simulink model "MobileRobotController"  (R2021b)
settings: Solver=VariableStepAuto  StartTime=0.0  StopTime=10.0  RelTol=1e-3
libraries: mobileRoboticsLib x3
settings Model: Creator=EarthPhisek  LastModifiedBy=EarthPhisek

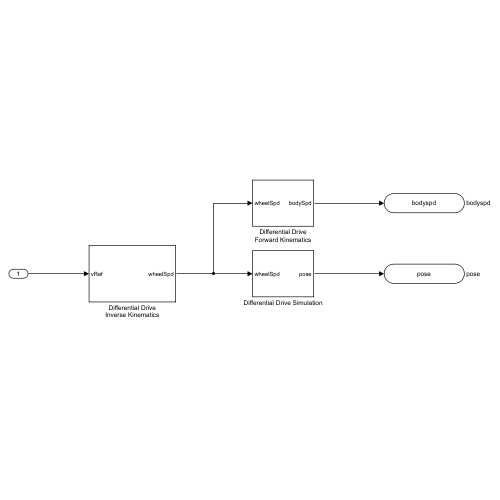
[thumbnail: Simulink's stored preview of the top-level diagram]
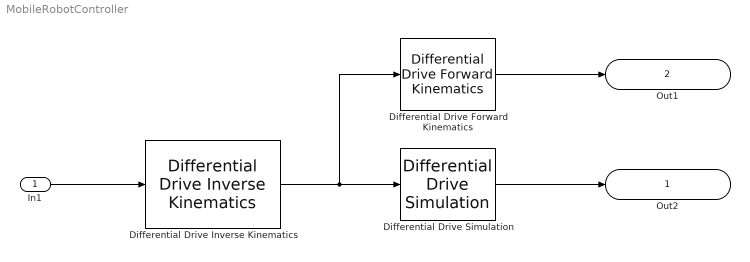
== system MobileRobotController ==
  In1 : Inport
  Differential Drive Forward Kinematics : mobileRoboticsLib/Kinematic Models/Differential Drive/Differential Drive Forward Kinematics  wheelRadius=0.1  wheelBase=0.5
      settings: SourceProductName=Mobile Robotics Simulation Toolbox
  Differential Drive Inverse Kinematics : mobileRoboticsLib/Kinematic Models/Differential Drive/Differential Drive Inverse Kinematics  wheelRadius=0.1  wheelBase=0.5
      settings: SourceProductName=Mobile Robotics Simulation Toolbox
  Differential Drive Simulation : mobileRoboticsLib/Kinematic Models/Differential Drive/Differential Drive Simulation  wheelRadius=0.1  wheelBase=0.5  initX=0  initY=0  initAngle=0  Ts=0.05
      settings: SourceProductName=Mobile Robotics Simulation Toolbox
  Out2 : Outport  SignalName=pose
  Out1 : Outport  Port=2  SignalName=bodyspd
  wires:
  Differential Drive Inverse Kinematics/1 -> Differential Drive Forward Kinematics/1, Differential Drive Simulation/1
  In1/1 -> Differential Drive Inverse Kinematics/1
  Differential Drive Forward Kinematics/1 -> Out1/1
  Differential Drive Simulation/1 -> Out2/1
